simulink model "positive"  (Simulink 8.5)
settings: Solver=ode15s  SolverMode=SingleTasking  StartTime=0.0  StopTime=0.5  FixedStep=0.06  RelTol=1e-3  AbsTol=1e-6
libraries: powerlib x27
settings Model: Creator=Dr. Lotfifard  LastModifiedBy=PC
settings DataIOCC: LimitDataPoints=off
settings OptimizationCC: BlockReduction=off  BooleanDataType=off
settings DebuggingCC: SaveWithParameterizedLinksMsg=none  SignalResolutionControl=TryResolveAllWithWarning  MultiTaskDSMMsg=warning  MultiTaskCondExecSysMsg=none  FcnCallInpInsideContextMsg=UseLocalSettings
settings HardwareCC: TargetUnknown=on

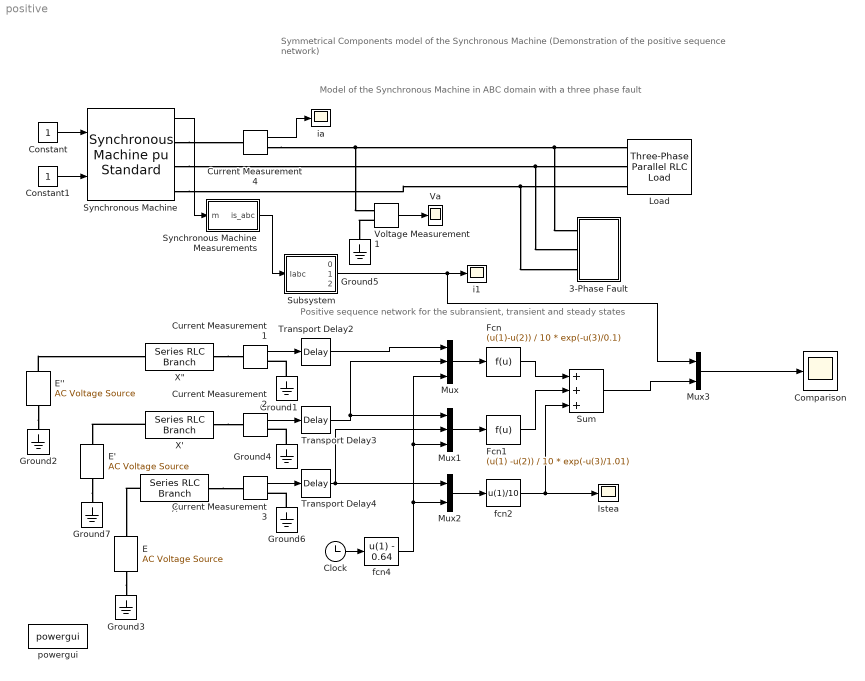
== system positive ==
  note: Symmetrical Components model of the Synchronous Machine
      | (Demonstration of the positive sequence network)
  note: Positive sequence network for the subransient, transient and steady states
  note: Model of the Synchronous Machine in ABC domain with a three phase fault
  3-Phase Fault : Subsystem  mask(3-Phase Fault){FaultTime=0.64}
      mask init:
      | 0.5
      mask Display: plot(0,0,100,100,[40,40,57,35,51],[20,5,73,48,95],[40,51],[5,20])
  Clock : Clock
  Comparison : Scope
      settings: TickLabels=on  TimeRange=3  YMin=-4  YMax=4  SaveName=vf
  Constant : Constant
  Constant1 : Constant
  Current Measurement{1..4} (4 alike) : powerlib/Measurements/Current Measurement  PhasorSimulation=off  OutputType=Complex  PSBequivalent=0
  E : powerlib/Electrical Sources/AC Voltage Source  Amplitude=100  Phase=0  Frequency=60  SampleTime=0  Measurements=None
  E' : powerlib/Electrical Sources/AC Voltage Source  Amplitude=100  Phase=0  Frequency=60  SampleTime=0  Measurements=None
  E'' : powerlib/Electrical Sources/AC Voltage Source  Amplitude=100  Phase=0  Frequency=60  SampleTime=0  Measurements=None
  Fcn : Fcn  Expr=(u(1)-u(2)) / 10 * exp(-u(3)/0.1)
  Fcn1 : Fcn  Expr=(u(1) -u(2)) / 10 * exp(-u(3)/1.01)
  Ground{1..7} (7 alike) : powerlib/Elements/Ground  LConnTagsString=a
  Istea : Scope
      settings: TickLabels=on  YMin=-1  YMax=1  SaveName=is
  Load : powerlib/Elements/Three-Phase Parallel RLC Load  LConnTagsString=A|B|C  Configuration=Y (grounded)  NominalVoltage=400*sqrt(3)  NominalFrequency=60  ActivePower=1  InductivePower=6000  CapacitivePower=0  Measurements=None  LoadType=constant Z
  Mux : Mux  Inputs=3
      settings: DisplayOption=signals
  Mux1 : Mux  Inputs=3
      settings: DisplayOption=signals
  Mux2 : Mux  Inputs=2
      settings: DisplayOption=signals
  Mux3 : Mux  Inputs=2
      settings: DisplayOption=signals
  Subsystem : Subsystem
  Sum : Sum  Inputs=+++  SaturateOnIntegerOverflow=on  InputSameDT=on  OutDataTypeStr=Inherit: Same as first input
  Synchronous Machine Measurements : Subsystem  mask(Synchronous Machine measurements){v1=on, v2=off, v3=off, v4=off, v5=off, v6=off, v7=off, v8=off, v9=off, v10=off}
      mask prompts: v1 "is_abc: stator currents (abc reference frame)"; v2 "is_qd: stator currents (qd reference frame)"; v3 "ifd: field current (qd reference frame)"; v4 "ik_qd: damper winding currents (qd reference frame)"; v5 "phim_qd: mutual fluxes (qd reference frame)"; v6 "vs_qd: stator voltages (qd reference frame)"; v7 "theta: rotor angular position"; v8 "N: rotor angular speed"; v9 "Pe: electrical power"; v10 "dw: rotor speed deviation"
      mask help:
      | Select the signals you want to observe.
      |
      | CAUTION: damper winding currents are referred to the stator.
      mask init:
      | s=[v1 v2 v3 v4 v5 v6 v7 v8 v9 v10];
      | laststate=str2num(get_param([gcb,'/last state'],'Value')); % last dialog box state
      | set_param([gcb,'/last state'],'Value',['[ ',num2str(s),' ]']);
      | 
      | if (sum(abs(laststate-s))) % if actual mask differs from last value
      |   % Name of output ports which reflect Synchronous Machine outputs
      |   names = {'is_abc','is_qd','ifd','ik_qd','phim_qd','vs_qd','theta','N','Pe','dw'};
      | 
      |   % Position of output ports for neat presentation
      |   positions = [ 145    54   165    66
      |               145    89   165   101
      |               145   124   165   136
      |               145   159   165   171
      |               145   194   165   206
      |               145   229   165   241
      |               145   264   165   276
      |               145   299   165   311
      |               145   334   165   346
      |               145   369   165   381
      |             ];
      |   % find_system options differ from ver5.0 to 5.1
      |   ver=version; ver=ver(1:3);
      | 
      |   % erase all existing outports to keep same order all the time
      |   for (i=1:length(s))
      |     switch(ver)
      |       case{'5.1'}
      |         if ~isempty(find_system(gcb,'LookUnderMasks','on','Name',names{i}))
      |           delete_line(gcb,['Demux/',num2str(i)],[names{i},'/1']);
      |           delete_block([gcb,'/',names{i}]);
      |         end	% if
      |       case{'5.0'}
      |         if ~isempty(find_system(gcb,'Name',names{i}))
      |           delete_line(gcb,['Demux/',num2str(i)],[names{i},'/1']);
      |           delete_block([gcb,'/',names{i}]);
      |         end	% if
      |     end % switch
      |   end % for
      | 
      |   % find outports desired
      |   idx=find(s~=0);
      | 
      |   for (i=idx)
      |     add_block('built-in/Outport',[gcb,'/',names{i}],'Position',positions(i,:));
      |     add_line(gcb,['Demux/',num2str(i)],[names{i},'/1']);
      |   end % for
      | end % if
  Synchronous Machine : powerlib/Machines/Synchronous Machine pu Standard  Tag=PoWeRsYsTeMbLoCk  PresetModel=No  MechanicalLoad=Mechanical power Pm  ShowDetailedParameters=on  RotorType=Salient-pole  Units=per unit standard parameters  MeasurementBus=off  NominalParameters="[ 187E6  13800   60]"  Reactances1=[ 1.81, 0.3, 0.23, 1.76, 0.65, 0.25, 0.15 ]  Reactances2="[ 1.305, 0.296, 0.252, 0.474,  0.243,  0.18 ]"  dAxisTimeConstants=Open-circuit  qAxisTimeConstants=Short-circuit  TimeConstants1="[ 4.4849  0.0681  0.1  ]"  TimeConstants2=[ 8.0, 0.03, 1.0, 0.07 ]  TimeConstants3="[  4.49  0.0681  0.0513  ]"  TimeConstants4=[ 8.0, 0.03, 0.3371, 0.0295 ]  TimeConstants5=[ 1.01, 0.053, 0.1 ]  TimeConstants6=[ 1.3201, 0.023, 1.0, 0.07 ]  TimeConstants7=[0.012 0.003 0.003]  TimeConstants8=[ 1.3201, 0.0231, 0.3371, 0.0295 ]  StatorResistance=0.003  Mechanical=[ 3.7 0 20 ]  PolePairs=20  InitialConditions="[ 0  0  0  0  0  0  0  0  1 ]"  SetSaturation=off  Saturation=[0.6404,0.7127,0.8441,0.9214,0.9956,1.082,1.19,1.316,1.457;0.7,0.7698,0.8872,0.9466,0.9969,1.046,1.1,1.151,1.201]  LoadFlowParameters=[1,0,0,0,0]  TsPowergui=0  TsBlock=-1  IterativeModel=Forward Euler  BusType=PV  Pref=0  Qref=0  Qmin=-inf  Qmax=inf  PLF=0  QLF=0
  Transport Delay2 : TransportDelay  DelayTime=0.64
  Transport Delay3 : TransportDelay  DelayTime=0.64
  Transport Delay4 : TransportDelay  DelayTime=0.64
  Va : Scope
      settings: TickLabels=on  TimeRange=3  YMin=-600  YMax=550  SaveName=vf
  Voltage Measurement1 : powerlib/Measurements/Voltage Measurement  PhasorSimulation=off  OutputType=Complex  PSBequivalent=0
  X : powerlib/Elements/Series RLC Branch  LConnTagsString=__new0  RConnTagsString=__new0  BranchType=RLC  Resistance=1  Inductance=1e-3  SetiL0=off  InitialCurrent=0  Capacitance=1e-6  Setx0=off  InitialVoltage=0  Measurements=None
  "X\"" : powerlib/Elements/Series RLC Branch  LConnTagsString=__new0  RConnTagsString=__new0  BranchType=RLC  Resistance=1  Inductance=1e-3  SetiL0=off  InitialCurrent=0  Capacitance=1e-6  Setx0=off  InitialVoltage=0  Measurements=None
  X' : powerlib/Elements/Series RLC Branch  LConnTagsString=__new0  RConnTagsString=__new0  BranchType=RLC  Resistance=1  Inductance=1e-3  SetiL0=off  InitialCurrent=0  Capacitance=1e-6  Setx0=off  InitialVoltage=0  Measurements=None
  fcn2 : Fcn  Expr=u(1)/10
  fcn4 : Fcn  Expr=u(1) - 0.64
  i1 : Scope
      settings: TickLabels=on  YMin=-2.5  YMax=2.5  SaveName=is
  ia : Scope
      settings: TickLabels=on  YMin=-100  YMax=15  SaveName=is
  powergui : powerlib/powergui  SimulationMode=Continuous  SolverType=Tustin/Backward Euler (TBE)  SampleTime=0  frequency=60  SPID=off  DisableSnubberDevices=off  DisableRonSwitches=off  DisableVfSwitches=off  SwTol=0  DisplayEquations=off  Interpol=off  methode=off  Ts=0  FunctionMessages=off  echomessages=off  HookPort=off  EnableUseOfTLC=off  x0status=blocks  frequencyindice=60  Pbase=100e6  ErrMax=1e-4  Iterations=50  UnitsV=kV  UnitsW=MW  buscounter=0  RestoreLinks=warning  ResistiveCurrentMeasurement=off  Frange=[0:2:500]  Ylog=off  Xlog=on  ShowGrid=off  save=off  variable=ZData  structure=0  ZoomFFT=on  StartTime=0.0  cycles=1  DisplayStyle=1  fundamental=60  FreqAxis=off  MaxFrequency=1000  frequencyindicesteady=1  RmsSteady=1  display=off
  wires:
  Current Measurement4/1 -> ia/1
  Voltage Measurement1/1 -> Va/1
  Subsystem/2(1) -> Mux3/1, i1/1
  Synchronous Machine Measurements/1(is_abc) -> Subsystem/1(Iabc)
  Mux/1 -> Fcn/1
  Mux1/1 -> Fcn1/1
  Transport Delay3/1 -> Mux1/1, Mux/2
  Fcn1/1 -> Sum/2
  fcn2/1 -> Istea/1, Sum/3
  Mux3/1 -> Comparison/1
  Sum/1 -> Mux3/2
  Clock/1 -> fcn4/1
  fcn4/1 -> Mux2/2, Mux/3, Mux1/3
  Transport Delay2/1 -> Mux/1
  Fcn/1 -> Sum/1
  Transport Delay4/1 -> Mux2/1, Mux1/2
  Constant/1 -> Synchronous Machine/1
  Constant1/1 -> Synchronous Machine/2
  Synchronous Machine/1 -> Synchronous Machine Measurements/1(m)
  Current Measurement1/1 -> Transport Delay2/1
  Current Measurement2/1 -> Transport Delay3/1
  Current Measurement3/1 -> Transport Delay4/1
  Mux2/1 -> fcn2/1
  connections:
  Voltage Measurement1/LConn2 -- Ground5/LConn1
  Current Measurement4/RConn1 -- Load/LConn1 -- 3-Phase Fault/LConn1 -- Voltage Measurement1/LConn1
  Synchronous Machine/RConn2 -- Load/LConn2 -- 3-Phase Fault/LConn2
  Synchronous Machine/RConn3 -- Load/LConn3 -- 3-Phase Fault/LConn3
  Synchronous Machine/RConn1 -- Current Measurement4/LConn1
  Ground1/LConn1 -- Current Measurement1/RConn1
  Ground4/LConn1 -- Current Measurement2/RConn1
  Ground6/LConn1 -- Current Measurement3/RConn1
  X/RConn1 -- Current Measurement3/LConn1
  X'/RConn1 -- Current Measurement2/LConn1
  "X\""/RConn1 -- Current Measurement1/LConn1
  E''/LConn1 -- Ground2/LConn1
  E/LConn1 -- Ground3/LConn1
  E'/LConn1 -- Ground7/LConn1
  E''/RConn1 -- "X\""/LConn1
  X'/LConn1 -- E'/RConn1
  X/LConn1 -- E/RConn1

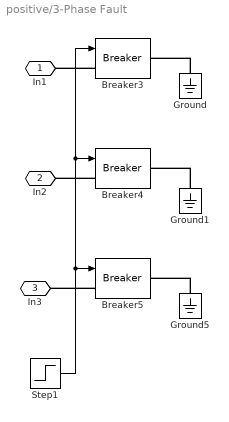
== system positive/3-Phase Fault ==
  Breaker3 : powerlib/Elements/Breaker  InitialState=0  SwitchingTimes="[ 1/60  5/60 ]"  External=on  BreakerResistance=0.01  SnubberResistance=1e6  SnubberCapacitance=inf  Measurements=None  MoreParameters=off  NoBreakLoop=off
  Breaker4 : powerlib/Elements/Breaker  InitialState=0  SwitchingTimes="[ 1/60  5/60 ]"  External=on  BreakerResistance=0.01  SnubberResistance=1e6  SnubberCapacitance=inf  Measurements=None  MoreParameters=off  NoBreakLoop=off
  Breaker5 : powerlib/Elements/Breaker  InitialState=0  SwitchingTimes="[ 1/60  5/60 ]"  External=on  BreakerResistance=0.01  SnubberResistance=1e6  SnubberCapacitance=inf  Measurements=None  MoreParameters=off  NoBreakLoop=off
  Ground : powerlib/Elements/Ground  LConnTagsString=a
  Ground1 : powerlib/Elements/Ground  LConnTagsString=a
  Ground5 : powerlib/Elements/Ground  LConnTagsString=a
  Step1 : Step  Time=FaultTime
  In1 : PMIOPort  Port=1  Side=Left
  In2 : PMIOPort  Port=2  Side=Left
  In3 : PMIOPort  Port=3  Side=Left
  wires:
  Step1/1 -> Breaker5/1, Breaker3/1, Breaker4/1
  connections:
  Breaker3/LConn1 -- In1/RConn1
  Breaker4/LConn1 -- In2/RConn1
  Breaker5/LConn1 -- In3/RConn1
  Ground5/LConn1 -- Breaker5/RConn1
  Ground1/LConn1 -- Breaker4/RConn1
  Ground/LConn1 -- Breaker3/RConn1

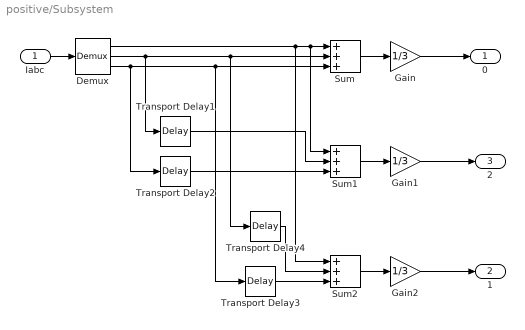
== system positive/Subsystem ==
  Iabc : Inport
  Demux : Demux  Outputs=3
  Gain : Gain  Gain=1/3  SaturateOnIntegerOverflow=on  OutDataTypeStr=Inherit: Same as input  ParamDataTypeStr=Inherit: Same as input
  Gain1 : Gain  Gain=1/3  SaturateOnIntegerOverflow=on  OutDataTypeStr=Inherit: Same as input  ParamDataTypeStr=Inherit: Same as input
  Gain2 : Gain  Gain=1/3  SaturateOnIntegerOverflow=on  OutDataTypeStr=Inherit: Same as input  ParamDataTypeStr=Inherit: Same as input
  Sum : Sum  Inputs=+++  SaturateOnIntegerOverflow=on  InputSameDT=on  OutDataTypeStr=Inherit: Same as first input
  Sum1 : Sum  Inputs=+++  SaturateOnIntegerOverflow=on  InputSameDT=on  OutDataTypeStr=Inherit: Same as first input
  Sum2 : Sum  Inputs=+++  SaturateOnIntegerOverflow=on  InputSameDT=on  OutDataTypeStr=Inherit: Same as first input
  Transport Delay1 : TransportDelay  DelayTime=1/(3*60)
  Transport Delay2 : TransportDelay  DelayTime=2/(3*60)
  Transport Delay3 : TransportDelay  DelayTime=1/(3*60)
  Transport Delay4 : TransportDelay  DelayTime=2/(3*60)
  0 : Outport  InitialOutput=0
  1 : Outport  Port=2  InitialOutput=0
  2 : Outport  Port=3  InitialOutput=0
  wires:
  Demux/2 -> Transport Delay1/1, Sum/2, Transport Delay4/1
  Transport Delay1/1 -> Sum1/2
  Transport Delay2/1 -> Sum1/3
  Transport Delay4/1 -> Sum2/2
  Demux/3 -> Transport Delay2/1, Sum/3, Transport Delay3/1
  Demux/1 -> Sum2/1, Sum/1, Sum1/1
  Transport Delay3/1 -> Sum2/3
  Iabc/1 -> Demux/1
  Sum/1 -> Gain/1
  Gain/1 -> 0/1
  Sum1/1 -> Gain1/1
  Gain1/1 -> 2/1
  Sum2/1 -> Gain2/1
  Gain2/1 -> 1/1

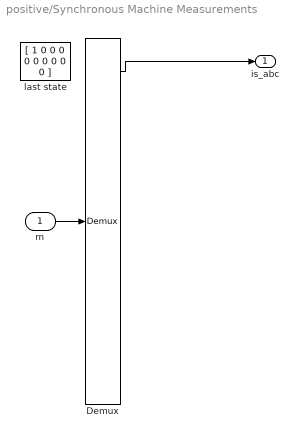
== system positive/Synchronous Machine Measurements ==
  m : Inport
  Demux : Demux  Outputs=[3,12,6,1,1,1]
  last state : Constant  Value="[ 1  0  0  0  0  0  0  0  0  0 ]"
  is_abc : Outport  InitialOutput=0
  wires:
  m/1 -> Demux/1
  Demux/1 -> is_abc/1
